simulink model "task11"  (R2014a)
settings: Solver=ode3  SolverMode=SingleTasking  StartTime=0.0  StopTime=20.0  FixedStep=0.5  RelTol=1e-3
InitFcn:
  | x = 1;
  | phi = 0;
  | theta = -19;
  | Atividade11 = readfis('Atividade11.fis');
libraries: fuzblock x1, simulink x1
settings Model: CovSFcnEnable=on  Creator=usuario  LastModifiedBy=User
settings OptimizationCC: BlockReduction=off  BooleanDataType=off
settings DebuggingCC: SaveWithParameterizedLinksMsg=none  UnderspecifiedInitializationDetection=Classic  SignalResolutionControl=TryResolveAllWithWarning  SolverPrmCheckMsg=none
settings HardwareCC: TargetUnknown=on

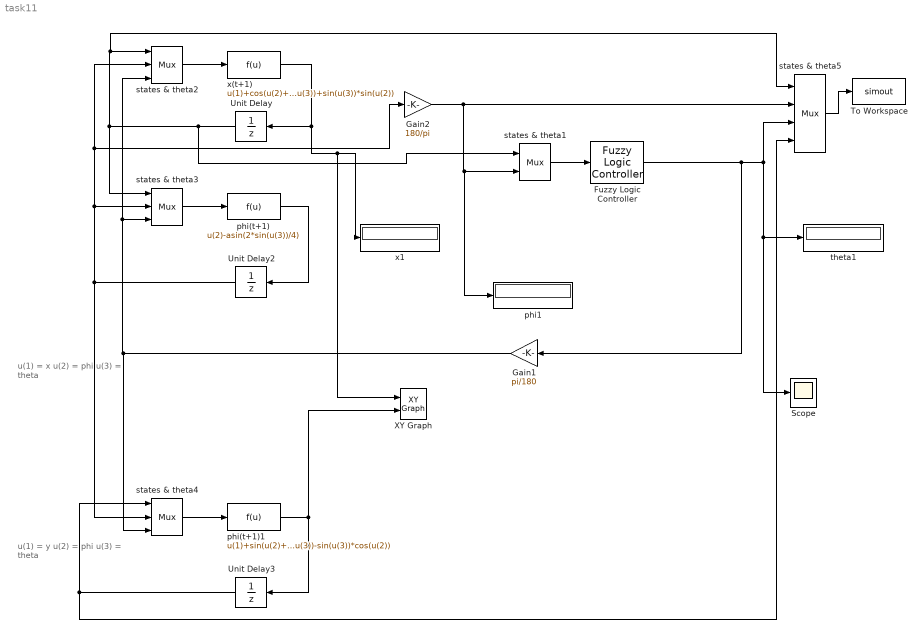
== system task11 ==
  note: u(1) = x
      | u(2) = phi
      | u(3) = theta
  note: u(1) = y
      | u(2) = phi
      | u(3) = theta
  Fuzzy Logic Controller : fuzblock/Fuzzy Logic  Controller  fis='Atividade11.fis'
  Gain1 : Gain  Gain=pi/180
  Gain2 : Gain  Gain=180/pi
  Scope : Scope
  To Workspace : ToWorkspace  VariableName=simout  SaveFormat=Timeseries  SampleTime=-1
  Unit Delay : UnitDelay  InitialCondition=13  SampleTime=-1
  Unit Delay2 : UnitDelay  InitialCondition=30*pi/180  SampleTime=-1
  Unit Delay3 : UnitDelay  InitialCondition=5  SampleTime=-1
  XY Graph : simulink/Sinks/XY Graph  xmin=0  xmax=15  ymin=0  ymax=30  st=-1
  phi(t+1) : Fcn  Expr=u(2)-asin(2*sin(u(3))/4)
  phi(t+1)1 : Fcn  Expr=u(1)+sin(u(2)+u(3))-sin(u(3))*cos(u(2))
  phi1 : Display
  states & theta1 : Mux  Inputs=2
  states & theta2 : Mux  Inputs=3
  states & theta3 : Mux  Inputs=3
  states & theta4 : Mux  Inputs=3
  states & theta5 : Mux
  theta1 : Display
  x(t+1) : Fcn  Expr=u(1)+cos(u(2)+u(3))+sin(u(3))*sin(u(2))
  x1 : Display
  wires:
  states & theta1/1 -> Fuzzy Logic Controller/1
  x(t+1)/1 -> Unit Delay/1, XY Graph/1, x1/1
  phi(t+1)/1 -> Unit Delay2/1
  states & theta2/1 -> x(t+1)/1
  states & theta3/1 -> phi(t+1)/1
  Fuzzy Logic Controller/1 -> Gain1/1, states & theta5/3, theta1/1, Scope/1
  Unit Delay/1 -> states & theta1/1, states & theta5/1, states & theta2/1, states & theta3/1
  Unit Delay2/1 -> states & theta4/2, states & theta3/2, Gain2/1, states & theta2/2
  phi(t+1)1/1 -> XY Graph/2, Unit Delay3/1
  states & theta4/1 -> phi(t+1)1/1
  Unit Delay3/1 -> states & theta5/4, states & theta4/1
  states & theta5/1 -> To Workspace/1
  Gain2/1 -> states & theta5/2, phi1/1, states & theta1/2
  Gain1/1 -> states & theta4/3, states & theta2/3, states & theta3/3
